simulink model "NED_to_ECEF"  (R2014a)
settings: Solver=ode45  StartTime=0.0  StopTime=orbit_period  RelTol=1e-3
values from neighbouring files (symbols this model uses):
  altitude = 405000    [Satellite_Setup_Sun_Pointing (1).m]    (also in Satellite_Setup_Sun_Pointing.m; Satellite_setup_ZenithPointing (1).m; Satellite_setup_ZenithPointing.m)
  igrf_L = 10    [Satellite_Setup_Sun_Pointing (1).m]    (also in Satellite_Setup_Sun_Pointing.m; Satellite_setup_ZenithPointing (1).m; Satellite_setup_ZenithPointing.m)
  igrf_tol = 1e-9    (= 1e-09)    [Satellite_Setup_Sun_Pointing (1).m]    (also in Satellite_Setup_Sun_Pointing.m; Satellite_setup_ZenithPointing (1).m; Satellite_setup_ZenithPointing.m)
undefined symbols (not defined in the file or in its folder): igrf_G, igrf_H
libraries: aerolibgravity2 x1, simulink x1
settings Model: Creator=Daire  LastModifiedBy=Daire

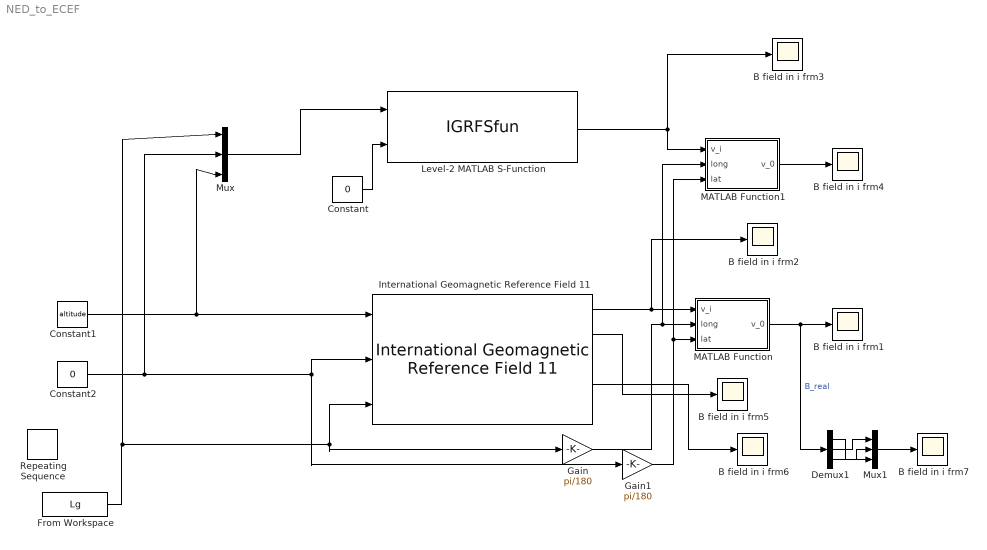
== system NED_to_ECEF ==
  B field in i frm{1..7} (7 alike) : Scope
      B field in i frm1 settings: YMin=-10000  YMax=35000  SaveName=ScopeData19
      B field in i frm2 settings: YMin=-15000  YMax=35000
      B field in i frm3 settings: YMin=-4e-05  YMax=6e-05
      B field in i frm4 settings: YMin=-2.25e-05  YMax=1.25e-05  SaveName=ScopeData2
      B field in i frm5 settings: YMin=21000  YMax=33000  SaveName=ScopeData3
      B field in i frm6 settings: YMin=-30  YMax=25  SaveName=ScopeData4
      B field in i frm7 settings: YMin=-10000  YMax=35000  SaveName=ScopeData5
  Constant : Constant  Value=0
  Constant1 : Constant  Value=altitude
  Constant2 : Constant  Value=0
  Demux1 : Demux  Outputs=3
  From Workspace : FromWorkspace  VariableName=Lg  SampleTime=0
  Gain : Gain  Gain=pi/180
  Gain1 : Gain  Gain=pi/180
  International Geomagnetic Reference Field 11 : aerolibgravity2/International Geomagnetic Reference Field 11  units=Metric (MKS)  time_in=off  month=February  day=1  year=2014  action=Error  sv_out=off
  Level-2 MATLAB S-Function : M-S-Function  FunctionName=IGRFSfun  Parameters=igrf_L,igrf_tol,igrf_G,igrf_H  mask{Parameter1=igrf_L, Parameter2=igrf_tol, Parameter3=igrf_G, Parameter4=igrf_H}
      mask prompts: Parameter1 "L"; Parameter2 "tolerance"; Parameter3 "G_coefs"; Parameter4 "H_coefs"
      mask Display:
      | disp('IGRF 11\n  Geomagnetic reference')
      | port_label('input',1,'LLA')
      | port_label('output',1,'real B')
  MATLAB Function : MATLAB Function  TreatAsAtomicUnit=on
  MATLAB Function1 : MATLAB Function  TreatAsAtomicUnit=on
  Mux : Mux  Inputs=3
  Mux1 : Mux  Inputs=3
  Repeating Sequence : simulink/Sources/Repeating Sequence  rep_seq_t=[0 5.547634839472084e+03]  rep_seq_y=[-180 180]
  wires:
  Constant2/1 -> Mux/2, International Geomagnetic Reference Field 11/2, Gain1/1
  Constant1/1 -> Mux/3, International Geomagnetic Reference Field 11/1
  From Workspace/1 -> Mux/1, International Geomagnetic Reference Field 11/3, Gain/1
  International Geomagnetic Reference Field 11/1 -> B field in i frm2/1, MATLAB Function/1(v_i)
  Gain/1 -> MATLAB Function1/2(long), MATLAB Function/2(long)
  Gain1/1 -> MATLAB Function1/3(lat), MATLAB Function/3(lat)
  Constant/1 -> Level-2 MATLAB S-Function/2
  Mux/1 -> Level-2 MATLAB S-Function/1
  Level-2 MATLAB S-Function/1 -> B field in i frm3/1, MATLAB Function1/1(v_i)
  MATLAB Function1/1(v_0) -> B field in i frm4/1
  International Geomagnetic Reference Field 11/2 -> B field in i frm5/1
  International Geomagnetic Reference Field 11/4 -> B field in i frm6/1
  Demux1/1 -> Mux1/3
  Demux1/2 -> Mux1/1
  MATLAB Function/1(v_0) -> Demux1/1, B field in i frm1/1  "B_real"
  Demux1/3 -> Mux1/2
  Mux1/1 -> B field in i frm7/1

== matlab function NED_to_ECEF/MATLAB Function1 ==
  data: v_i input; v_0 output; long input; lat input
function v_0 = NED_to_ECEF(v_i,long,lat)
%#codegen
 
lat=(pi/2)-lat;

R=[-sin(lat)*cos(long), -sin(long), -cos(lat)*cos(long);...
    -sin(lat)*sin(long), cos(long), -cos(lat)*sin(long);...
    cos(lat), 0, -sin(lat)];

v_0=R*v_i;

end

== matlab function NED_to_ECEF/MATLAB Function ==
  data: v_i input; v_0 output; long input; lat input
function v_0 = NED_to_ECEF(v_i,long,lat)
%#codegen
 
%lat=(pi/2)-lat;

R=[-sin(lat)*cos(long), -sin(long), -cos(lat)*cos(long);...
    -sin(lat)*sin(long), cos(long), -cos(lat)*sin(long);...
    cos(lat), 0, -sin(lat)];

v_0=R*v_i;

end
